simulink model "path_following"  (R2022b)
settings: Solver=VariableStepAuto  StartTime=0.0  StopTime=10.0  RelTol=1e-3
settings Model: Creator=XinyiWu  LastModifiedBy=XinyiWu

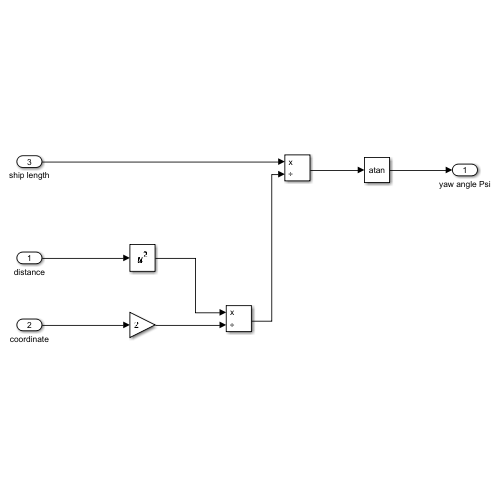
[thumbnail: Simulink's stored preview of the top-level diagram]
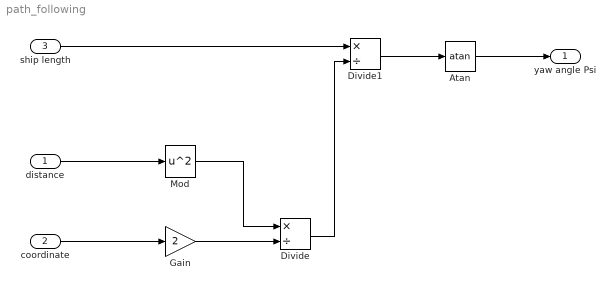
== system path_following ==
  distance : Inport
  coordinate : Inport  Port=2
  ship length : Inport  Port=3
  Atan : Trigonometry  Operator=atan
  Divide : Product  Inputs=*/
  Divide1 : Product  Inputs=*/
  Gain : Gain  Gain=2
  Mod : Math  Operator=square
  yaw angle Psi : Outport
  wires:
  distance/1 -> Mod/1
  coordinate/1 -> Gain/1
  Mod/1 -> Divide/1
  Gain/1 -> Divide/2
  ship length/1 -> Divide1/1
  Divide/1 -> Divide1/2
  Divide1/1 -> Atan/1
  Atan/1 -> yaw angle Psi/1
